simulink model "kiLicopter_openloop2"  (R2025b)
settings: Solver=ode45  StartTime=0.0  StopTime=17.8  MaxStep=0.1  RelTol=1e-3
settings Model: Creator=MTMTAD006  LastModifiedBy=MTMTAD006

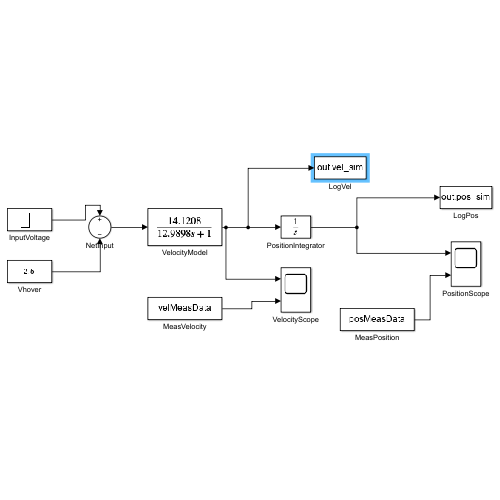
[thumbnail: Simulink's stored preview of the top-level diagram]
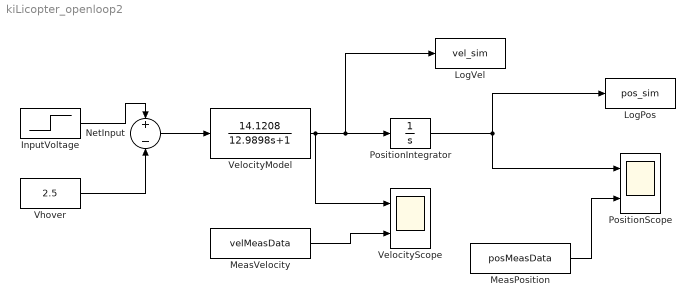
== system kiLicopter_openloop2 ==
  InputVoltage : Step  Time=0  Before=2.5  After=5  SampleTime=0
  LogPos : ToWorkspace  VariableName=pos_sim  SaveFormat=Timeseries  SampleTime=-1
  LogVel : ToWorkspace  VariableName=vel_sim  SaveFormat=Timeseries  SampleTime=-1
  MeasPosition : FromWorkspace  VariableName=posMeasData  OutputAfterFinalValue=Holding final value
  MeasVelocity : FromWorkspace  VariableName=velMeasData  OutputAfterFinalValue=Holding final value
  NetInput : Sum  Inputs=+-
  PositionIntegrator : Integrator
  PositionScope : Scope  NumInputPorts=2
  VelocityModel : TransferFcn  Numerator=14.1208  Denominator=[12.9898 1]
  VelocityScope : Scope  NumInputPorts=2
  Vhover : Constant  Value=2.5
  wires:
  InputVoltage/1 -> NetInput/1
  Vhover/1 -> NetInput/2
  NetInput/1 -> VelocityModel/1
  VelocityModel/1 -> PositionIntegrator/1, LogVel/1, VelocityScope/1
  MeasVelocity/1 -> VelocityScope/2
  PositionIntegrator/1 -> PositionScope/1, LogPos/1
  MeasPosition/1 -> PositionScope/2
